simulink model "FOPD_linear_model"  (Simulink 9.2)
settings: Solver=ode4  StartTime=0.0  StopTime=10.0  FixedStep=0.01  MaxStep=0.2  RelTol=1e-3
settings Model: Creator=standard  LastModifiedBy=standard
settings DataIOCC: LimitDataPoints=off  SaveFormat=Dataset  SignalLoggingSaveFormat=Dataset
settings OptimizationCC: LifeSpan=auto
settings DebuggingCC: UnderspecifiedInitializationDetection=Simplified  MergeDetectMultiDrivingBlocksExec=error  FcnCallInpInsideContextMsg=error  StateNameClashWarn=none  SFUnexpectedBacktrackingDiag=error  SFNoUnconditionalDefaultTransitionDiag=error  SFExecutionAtInitializationDiag=warning
settings HardwareCC: ProdBitPerPointer=64  ProdBitPerSizeT=64  ProdBitPerPtrDiffT=64  ProdLargestAtomicFloat=Float  ProdIntDivRoundTo=Zero  ProdEndianess=LittleEndian  ProdWordSize=64  ProdHWDeviceType=Intel->x86-64 (Windows64)
settings ModelReferenceCC: PropagateSignalLabelsOutOfModel=on
settings SFSimCC: SimUseLocalCustomCode=on
settings RTWCC: RTWUseLocalCustomCode=on
settings CodeAppCC: StateflowObjectComments=off
settings GRTTargetCC: TargetLangStandard=C99 (ISO)  GeneratePreprocessorConditionals=Use local settings  CombineOutputUpdateFcns=on  GRTInterface=off
settings ConfigComp: CovMetricSettings=dwe  CovHtmlReporting=off  CovSaveCumulativeToWorkspaceVar=off  CovSaveSingleToWorkspaceVar=off  CovExternalEMLEnable=on

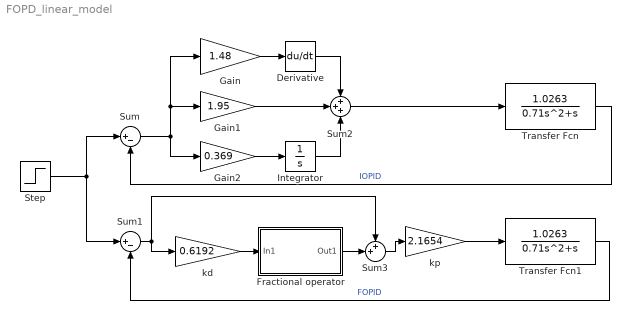
== system FOPD_linear_model ==
  Derivative : Derivative
  "Fractional operator " : Subsystem  mask{gam=1.0497, ww=[1e-3, 1e3], n=5, kF1=on, kF=Modified Oustaloup filter}
      mask prompts: gam "Derivative order gamma"; ww "Frequency range [wb,wh]"; n "Apprixmation order"; kF1 "Is a low-pass filter required?"; kF "Filter type"
      mask init:
      | wb=ww(1); wh=ww(2); 
      | if kF==1, G=ousta_fod(gam,n,wb,wh);
      | else, G=new_fod(gam,n,wb,wh); end
      | num=G.num{1}; den=G.den{1}; T=1/wh; str='Fractional\n';
      | MaskDescription=num;
      | if isnumeric(gam)
      | 	if gam>0, str=[str, 'Der  s^' num2str(gam) ];
      | 	else, str=[str, 'Int  s^{' num2str(gam) '}']; end
      | else, str=[str, 'Der  s^gam']; end
      | if kF1==1, G=G*tf(1,[T 1]); end
      mask TypeOptions kF: Oustaloup filter | Modified Oustaloup filter | Matsuda-Fujii filter
      mask DialogControl num_la Prompt: num_la
      mask Display: disp(str)
  Gain : Gain  Gain=1.48
  Gain1 : Gain  Gain=1.95
  Gain2 : Gain  Gain=0.369
  Integrator : Integrator
  Step : Step  SampleTime=0
  Sum : Sum  Inputs=|+-
  Sum1 : Sum  Inputs=|+-
  Sum2 : Sum  Inputs=+++
  Sum3 : Sum  Inputs=++|
  Transfer Fcn : TransferFcn  Numerator=[1.0263]  Denominator=[0.71 1 0]
  Transfer Fcn1 : TransferFcn  Numerator=[1.0263]  Denominator=[0.71 1 0]
  kd : Gain  Gain=0.6192
  kp : Gain  Gain=2.1654
  wires:
  Transfer Fcn/1 -> Sum/2  "IOPID"
  Step/1 -> Sum1/1, Sum/1
  Transfer Fcn1/1 -> Sum1/2  "FOPID"
  kp/1 -> Transfer Fcn1/1
  Gain/1 -> Derivative/1
  Gain2/1 -> Integrator/1
  Derivative/1 -> Sum2/1
  Integrator/1 -> Sum2/3
  Gain1/1 -> Sum2/2
  Sum/1 -> Gain1/1, Gain/1, Gain2/1
  Sum2/1 -> Transfer Fcn/1
  Sum1/1 -> Sum3/1, kd/1
  Sum3/1 -> kp/1
  "Fractional operator "/1(Out1) -> Sum3/2
  kd/1 -> "Fractional operator "/1(In1)

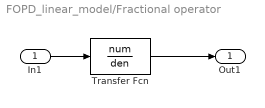
== system FOPD_linear_model/Fractional operator  ==
  In1 : Inport
  Transfer Fcn : TransferFcn  Numerator=num  Denominator=den
  Out1 : Outport
  wires:
  In1/1 -> Transfer Fcn/1
  Transfer Fcn/1 -> Out1/1
